simulink model "scmodel_4rw"  (R2022b)
settings: Solver=VariableStepAuto  StartTime=0.0  StopTime=100  RelTol=1e-3  AbsTol=1e-3
values from neighbouring files (symbols this model uses):
  N = 10    [quatshortpath.m]
  s = surf(xsphere, ysphere, zsphere)    [quatsphere.m]    (also in sphersphere.m; visualise.m = animatedline(rs_sta(1, 1), rs_sta(1, 2), rs_sta(1, 3), 'Colo; visualiseenv.m = surf(xsphere, ysphere, zsphere, 'DisplayName', 'Attitude Sph; visualisetraj.m = animatedline(rs_sta(1, 1), rs_sta(1, 2), rs_sta(1, 3), 'Colo)
  Z = 4e-4    (= 0.0004)    [test.m]
undefined symbols (not defined in the file or in its folder): X, Y
libraries: sm_lib x40, nesl_utility x37, matrix_library x3, dspsolvers x1
(part 2 of 2)

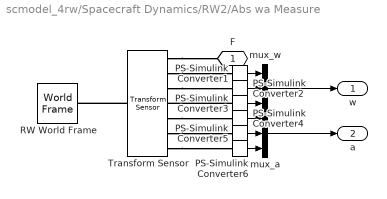
== system scmodel_4rw/Spacecraft Dynamics/RW2/Abs wa Measure ==
  PS-Simulink Converter{1..6} (6 alike) : nesl_utility/PS-Simulink Converter  PhysicalDomain=network_engine_domain  SubClassName=ps_output  LeftPortType=input  RightPortType=output  PseudoPeriodic=off  Frequencies=[]  VectorFormat=inherit  Unit=inherit  AffineConversion=off
  RW World Frame : sm_lib/Frames and Transforms/World Frame
  Transform Sensor : sm_lib/Frames and Transforms/Transform Sensor  MeasurementFrame=World  SenseAngle=off  SenseAxis=off  SenseQ=off  SenseR=off  SenseRotationSequence=off  RotationSequence=XYX  SenseOmegaX=on  SenseOmegaY=on  SenseOmegaZ=on  SenseQDot=off  SenseRDot=off  SenseAlphaX=on  SenseAlphaY=on  SenseAlphaZ=on  SenseQDDot=off  SenseRDDot=off  SenseX=off  SenseY=off  SenseZ=off  SenseRad=off  SenseAzim=off  SenseDist=off  SenseInc=off  SenseXDot=off  SenseYDot=off  SenseZDot=off  SenseRadDot=off  SenseAzimDot=off  SenseDistDot=off  SenseIncDot=off  SenseXDDot=off  SenseYDDot=off  SenseZDDot=off  SenseRadDDot=off  SenseAzimDDot=off  SenseDistDDot=off  SenseIncDDot=off
  mux_a : Mux  Inputs=3
  mux_w : Mux  Inputs=3
  F : PMIOPort  Side=Right
  w : Outport
  a : Outport  Port=2
  wires:
  mux_w/1 -> w/1
  PS-Simulink Converter5/1 -> mux_a/2
  PS-Simulink Converter2/1 -> mux_w/2
  PS-Simulink Converter3/1 -> mux_w/3
  PS-Simulink Converter1/1 -> mux_w/1
  mux_a/1 -> a/1
  PS-Simulink Converter6/1 -> mux_a/3
  PS-Simulink Converter4/1 -> mux_a/1
  connections:
  Transform Sensor/RConn7 -- PS-Simulink Converter6/LConn1
  Transform Sensor/RConn5 -- PS-Simulink Converter4/LConn1
  Transform Sensor/RConn2 -- PS-Simulink Converter1/LConn1
  PS-Simulink Converter3/LConn1 -- Transform Sensor/RConn4
  Transform Sensor/LConn1 -- RW World Frame/RConn1
  Transform Sensor/RConn6 -- PS-Simulink Converter5/LConn1
  Transform Sensor/RConn3 -- PS-Simulink Converter2/LConn1
  Transform Sensor/RConn1 -- F/RConn1

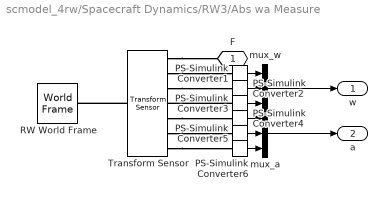
== system scmodel_4rw/Spacecraft Dynamics/RW3/Abs wa Measure ==
  PS-Simulink Converter{1..6} (6 alike) : nesl_utility/PS-Simulink Converter  PhysicalDomain=network_engine_domain  SubClassName=ps_output  LeftPortType=input  RightPortType=output  PseudoPeriodic=off  Frequencies=[]  VectorFormat=inherit  Unit=inherit  AffineConversion=off
  RW World Frame : sm_lib/Frames and Transforms/World Frame
  Transform Sensor : sm_lib/Frames and Transforms/Transform Sensor  MeasurementFrame=World  SenseAngle=off  SenseAxis=off  SenseQ=off  SenseR=off  SenseRotationSequence=off  RotationSequence=XYX  SenseOmegaX=on  SenseOmegaY=on  SenseOmegaZ=on  SenseQDot=off  SenseRDot=off  SenseAlphaX=on  SenseAlphaY=on  SenseAlphaZ=on  SenseQDDot=off  SenseRDDot=off  SenseX=off  SenseY=off  SenseZ=off  SenseRad=off  SenseAzim=off  SenseDist=off  SenseInc=off  SenseXDot=off  SenseYDot=off  SenseZDot=off  SenseRadDot=off  SenseAzimDot=off  SenseDistDot=off  SenseIncDot=off  SenseXDDot=off  SenseYDDot=off  SenseZDDot=off  SenseRadDDot=off  SenseAzimDDot=off  SenseDistDDot=off  SenseIncDDot=off
  mux_a : Mux  Inputs=3
  mux_w : Mux  Inputs=3
  F : PMIOPort  Side=Right
  w : Outport
  a : Outport  Port=2
  wires:
  mux_w/1 -> w/1
  PS-Simulink Converter5/1 -> mux_a/2
  PS-Simulink Converter2/1 -> mux_w/2
  PS-Simulink Converter3/1 -> mux_w/3
  PS-Simulink Converter1/1 -> mux_w/1
  mux_a/1 -> a/1
  PS-Simulink Converter6/1 -> mux_a/3
  PS-Simulink Converter4/1 -> mux_a/1
  connections:
  Transform Sensor/RConn7 -- PS-Simulink Converter6/LConn1
  Transform Sensor/RConn5 -- PS-Simulink Converter4/LConn1
  Transform Sensor/RConn2 -- PS-Simulink Converter1/LConn1
  PS-Simulink Converter3/LConn1 -- Transform Sensor/RConn4
  Transform Sensor/LConn1 -- RW World Frame/RConn1
  Transform Sensor/RConn6 -- PS-Simulink Converter5/LConn1
  Transform Sensor/RConn3 -- PS-Simulink Converter2/LConn1
  Transform Sensor/RConn1 -- F/RConn1

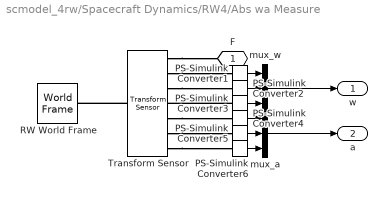
== system scmodel_4rw/Spacecraft Dynamics/RW4/Abs wa Measure ==
  PS-Simulink Converter{1..6} (6 alike) : nesl_utility/PS-Simulink Converter  PhysicalDomain=network_engine_domain  SubClassName=ps_output  LeftPortType=input  RightPortType=output  PseudoPeriodic=off  Frequencies=[]  VectorFormat=inherit  Unit=inherit  AffineConversion=off
  RW World Frame : sm_lib/Frames and Transforms/World Frame
  Transform Sensor : sm_lib/Frames and Transforms/Transform Sensor  MeasurementFrame=World  SenseAngle=off  SenseAxis=off  SenseQ=off  SenseR=off  SenseRotationSequence=off  RotationSequence=XYX  SenseOmegaX=on  SenseOmegaY=on  SenseOmegaZ=on  SenseQDot=off  SenseRDot=off  SenseAlphaX=on  SenseAlphaY=on  SenseAlphaZ=on  SenseQDDot=off  SenseRDDot=off  SenseX=off  SenseY=off  SenseZ=off  SenseRad=off  SenseAzim=off  SenseDist=off  SenseInc=off  SenseXDot=off  SenseYDot=off  SenseZDot=off  SenseRadDot=off  SenseAzimDot=off  SenseDistDot=off  SenseIncDot=off  SenseXDDot=off  SenseYDDot=off  SenseZDDot=off  SenseRadDDot=off  SenseAzimDDot=off  SenseDistDDot=off  SenseIncDDot=off
  mux_a : Mux  Inputs=3
  mux_w : Mux  Inputs=3
  F : PMIOPort  Side=Right
  w : Outport
  a : Outport  Port=2
  wires:
  mux_w/1 -> w/1
  PS-Simulink Converter5/1 -> mux_a/2
  PS-Simulink Converter2/1 -> mux_w/2
  PS-Simulink Converter3/1 -> mux_w/3
  PS-Simulink Converter1/1 -> mux_w/1
  mux_a/1 -> a/1
  PS-Simulink Converter6/1 -> mux_a/3
  PS-Simulink Converter4/1 -> mux_a/1
  connections:
  Transform Sensor/RConn7 -- PS-Simulink Converter6/LConn1
  Transform Sensor/RConn5 -- PS-Simulink Converter4/LConn1
  Transform Sensor/RConn2 -- PS-Simulink Converter1/LConn1
  PS-Simulink Converter3/LConn1 -- Transform Sensor/RConn4
  Transform Sensor/LConn1 -- RW World Frame/RConn1
  Transform Sensor/RConn6 -- PS-Simulink Converter5/LConn1
  Transform Sensor/RConn3 -- PS-Simulink Converter2/LConn1
  Transform Sensor/RConn1 -- F/RConn1

== matlab function scmodel_4rw/Controller/Controller ==
  data: Q_tar input; tau output; Q_cur input; Qd_cur input; ks input; ps input; v output; q output
function [tau, v, q]    = fcn(Q_tar, Q_cur, Qd_cur, ks, ps)  
    %convert from Q to Qm
    Qm_cur = quatconvert(Q_cur, 'simulink', 'matlab');
    Qm_tar = quatconvert(Q_tar, 'simulink', 'matlab');
    Qmd_cur = quatconvert(Qd_cur, 'simulink', 'matlab');
    Vmd_cur = rotvec(Qmd_cur);
    
    %find rotated versions of x, y, and z, and torques
    mn = size(ps);
    ps_cur = zeros(mn);
    ps_tar = zeros(mn);
    taus = zeros(mn);
    for i = 1:mn(1)
        ps_cur(i, :) = rotatepoint(Qm_cur, ps(i, :));
        ps_tar(i, :) = rotatepoint(Qm_tar, ps(i, :));
        taus(i, :) = cross(ps_cur(i, :), ks(i) * (ps_tar(i, :) - ps_cur(i, :)));
    end
    v = ps_cur(1)
    q = ps_tar(1)
    
    %find torque
    tau = -1*sum(taus);

== matlab function scmodel_4rw/Path Planner ==
  data: t input; q_tar output
function q_tar = fcn(t)
    theta = pi;
    phi = 2*pi*t/100;
    V_theta = theta*[sin(phi), -cos(phi), 0];
    V_phi = phi*[0, 0, 1];
    qm_tar = quaternion(V_phi, 'rotvec') * quaternion(V_theta, 'rotvec');
    q_tar = quatconvert(qm_tar, 'matlab', 'simulink');
end
